simulink model "DHS_Direct_Control_PI"  (R2019b)
settings: Solver=VariableStepAuto  StartTime=0.0  StopTime=0.5  RelTol=1e-3
undefined symbols (not defined in the file): Apd_i_dhs, Apd_u_dhs, C_dhs, f_sw_dhs, L_dhs, Tid_i_dhs, Tid_u_dhs, U_DC
libraries: simulink x2
settings Model: Creator=kissd  LastModifiedBy=kissd

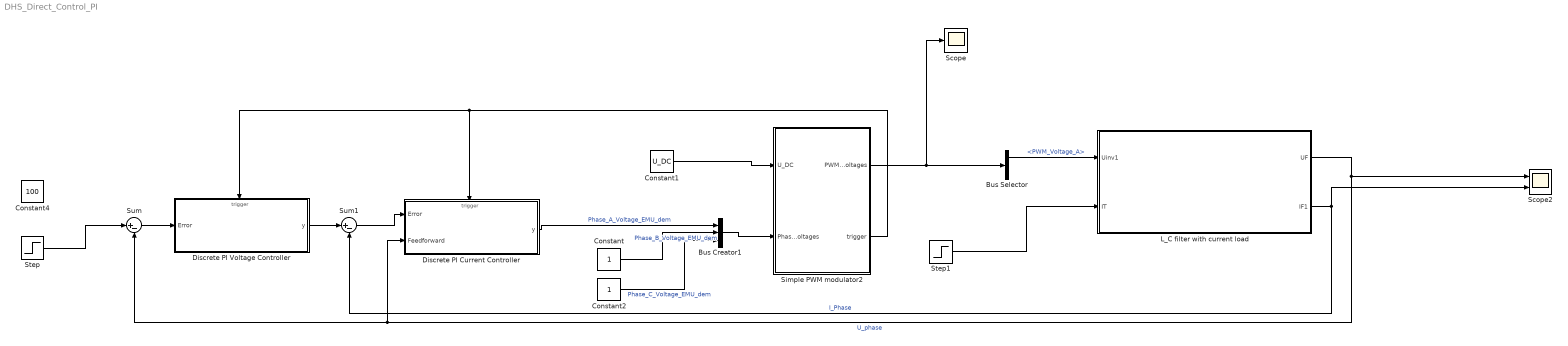
== system DHS_Direct_Control_PI ==
  Bus Creator1 : BusCreator  Inputs=3
  Bus Selector : BusSelector  OutputSignals=PWM_Voltage_A,PWM_Voltage_B,PWM_Voltage_C
  Constant : Constant
  Constant1 : Constant  Value=U_DC
  Constant2 : Constant
  Constant4 : Constant  Value=100
  Discrete PI Current Controller : Subsystem  AncestorBlock=controllers/Discrete PI Controller  mask(Continous PI Controller){Apd=Apd_i_dhs, Tid=Tid_i_dhs, fs=f_sw_dhs, UpperSat=U_DC, LowerSat=0}
      mask prompts: Apd "Proprotional Gain"; Tid "Integration Time"; fs "fsw"; UpperSat "Max. Saturation"; LowerSat "Min. Saturation"
      mask help: Continous PI Controller description.
  Discrete PI Voltage Controller : Subsystem  AncestorBlock=controllers/Discrete PI Controller  mask(Continous PI Controller){Apd=Apd_u_dhs, Tid=Tid_u_dhs, fs=f_sw_dhs, UpperSat=200, LowerSat=-200}
      mask prompts: Apd "Proprotional Gain"; Tid "Integration Time"; fs "fsw"; UpperSat "Max. Saturation"; LowerSat "Min. Saturation"
      mask help: Continous PI Controller description.
  L_C filter with current load : Subsystem
  Scope : Scope
  Scope2 : Scope  NumInputPorts=2
  Simple PWM modulator2 : Subsystem  AncestorBlock=controllers/Simple PWM modulator
  Step : Step  Time=0.2  Before=10  After=200  SampleTime=0
  Step1 : Step  Time=0.3  After=100  SampleTime=0
  Sum : Sum  Inputs=|+-
  Sum1 : Sum  Inputs=|+-
  wires:
  Simple PWM modulator2/2(trigger) -> Discrete PI Voltage Controller/Trigger, Discrete PI Current Controller/Trigger
  Discrete PI Current Controller/1(y) -> Bus Creator1/1  "Phase_A_Voltage_EMU_dem"
  Bus Creator1/1 -> Simple PWM modulator2/2(Phase_Voltages)
  Discrete PI Voltage Controller/1(y) -> Sum1/1
  Step/1 -> Sum/1
  Simple PWM modulator2/1(PWM_Voltages) -> Bus Selector/1, Scope/1
  Sum/1 -> Discrete PI Voltage Controller/1(Error)
  Constant/1 -> Bus Creator1/2  "Phase_B_Voltage_EMU_dem"
  Constant2/1 -> Bus Creator1/3  "Phase_C_Voltage_EMU_dem"
  L_C filter with current load/2(IF1) -> Scope2/2, Sum1/2  "I_Phase"
  L_C filter with current load/1(UF) -> Discrete PI Current Controller/2(Feedforward), Sum/2, Scope2/1  "U_phase"
  Bus Selector/1 -> L_C filter with current load/1(Uinv1)  "<PWM_Voltage_A>"
  Sum1/1 -> Discrete PI Current Controller/1(Error)
  Constant1/1 -> Simple PWM modulator2/1(U_DC)
  Step1/1 -> L_C filter with current load/2(IT)

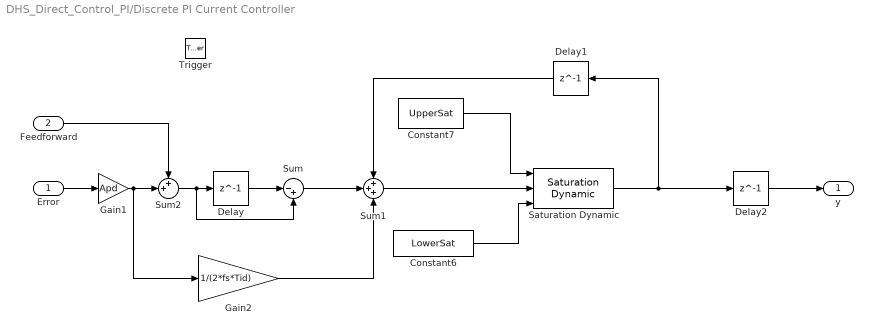
== system DHS_Direct_Control_PI/Discrete PI Current Controller ==
  Error : Inport
  Feedforward : Inport  Port=2
  Trigger : TriggerPort  TriggerType=either  VariantControl=Variant  PortDimensions=1
  Constant6 : Constant  Value=LowerSat
  Constant7 : Constant  Value=UpperSat
  Delay : Delay  DelayLength=1
  Delay1 : Delay  DelayLength=1
  Delay2 : Delay  DelayLength=1
  Gain1 : Gain  Gain=Apd
  Gain2 : Gain  Gain=1/(2*fs*Tid)
  Saturation Dynamic : simulink/Discontinuities/Saturation Dynamic  OutMin=[]  OutMax=[]  OutDataTypeStr=Inherit: Same as second input  OutDataType=fixdt(1, 16)  OutScaling=2^-10  DoSatur=off
  Sum : Sum  Inputs=|-+
  Sum1 : Sum  Inputs=+++
  Sum2 : Sum  Inputs=++|
  y : Outport
  wires:
  Error/1 -> Gain1/1
  Gain1/1 -> Sum2/2, Gain2/1
  Sum1/1 -> Saturation Dynamic/2
  Saturation Dynamic/1 -> Delay1/1, Delay2/1
  Constant7/1 -> Saturation Dynamic/1
  Constant6/1 -> Saturation Dynamic/3
  Delay/1 -> Sum/1
  Sum/1 -> Sum1/2
  Gain2/1 -> Sum1/3
  Delay1/1 -> Sum1/1
  Delay2/1 -> y/1
  Sum2/1 -> Sum/2, Delay/1
  Feedforward/1 -> Sum2/1

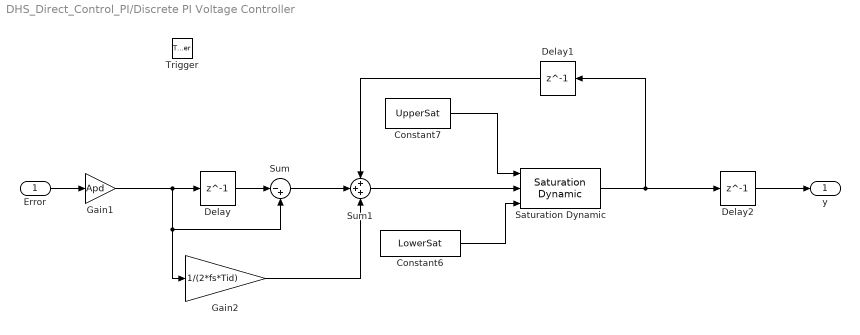
== system DHS_Direct_Control_PI/Discrete PI Voltage Controller ==
  Error : Inport
  Trigger : TriggerPort  TriggerType=either  VariantControl=Variant  PortDimensions=1
  Constant6 : Constant  Value=LowerSat
  Constant7 : Constant  Value=UpperSat
  Delay : Delay  DelayLength=1
  Delay1 : Delay  DelayLength=1
  Delay2 : Delay  DelayLength=1
  Gain1 : Gain  Gain=Apd
  Gain2 : Gain  Gain=1/(2*fs*Tid)
  Saturation Dynamic : simulink/Discontinuities/Saturation Dynamic  OutMin=[]  OutMax=[]  OutDataTypeStr=Inherit: Same as second input  OutDataType=fixdt(1, 16)  OutScaling=2^-10  DoSatur=off
  Sum : Sum  Inputs=|-+
  Sum1 : Sum  Inputs=+++
  y : Outport
  wires:
  Error/1 -> Gain1/1
  Gain1/1 -> Gain2/1, Sum/2, Delay/1
  Sum1/1 -> Saturation Dynamic/2
  Saturation Dynamic/1 -> Delay1/1, Delay2/1
  Constant7/1 -> Saturation Dynamic/1
  Constant6/1 -> Saturation Dynamic/3
  Delay/1 -> Sum/1
  Sum/1 -> Sum1/2
  Gain2/1 -> Sum1/3
  Delay1/1 -> Sum1/1
  Delay2/1 -> y/1

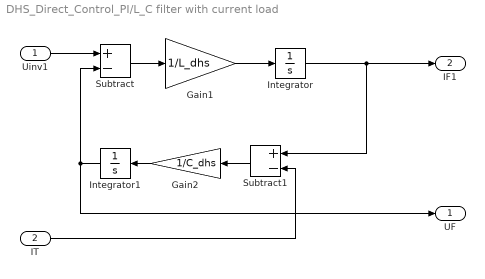
== system DHS_Direct_Control_PI/L_C filter with current load ==
  Uinv1 : Inport
  IT : Inport  Port=2
  Gain1 : Gain  Gain=1/L_dhs
  Gain2 : Gain  Gain=1/C_dhs
  Integrator : Integrator
  Integrator1 : Integrator
  Subtract : Sum  Inputs=+-
  Subtract1 : Sum  Inputs=+-
  UF : Outport
  IF1 : Outport  Port=2
  wires:
  Integrator1/1 -> UF/1, Subtract/2
  Subtract/1 -> Gain1/1
  Gain1/1 -> Integrator/1
  Integrator/1 -> Subtract1/1, IF1/1
  IT/1 -> Subtract1/2
  Gain2/1 -> Integrator1/1
  Uinv1/1 -> Subtract/1
  Subtract1/1 -> Gain2/1

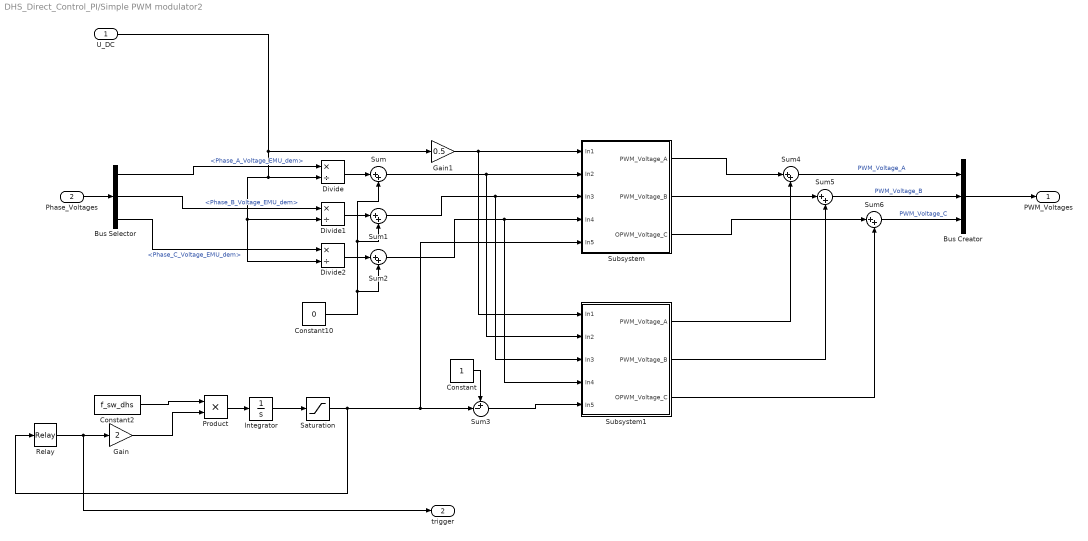
== system DHS_Direct_Control_PI/Simple PWM modulator2 ==
  U_DC : Inport
  Phase_Voltages : Inport  Port=2
  Bus Creator : BusCreator  Inputs=3
  Bus Selector : BusSelector  OutputSignals=Phase_A_Voltage_EMU_dem,Phase_B_Voltage_EMU_dem,Phase_C_Voltage_EMU_dem
  Constant : Constant
  Constant10 : Constant  Value=0
  Constant2 : Constant  Value=f_sw_dhs
  Divide : Product  Inputs=*/
  Divide1 : Product  Inputs=*/
  Divide2 : Product  Inputs=*/
  Gain : Gain  Gain=2
  Gain1 : Gain  Gain=0.5
  Integrator : Integrator
  Product : Product
  Relay : Relay  OnSwitchValue=1  OffSwitchValue=0  OnOutputValue=-1  OffOutputValue=1
  Saturation : Saturate  UpperLimit=1  LowerLimit=0
  Subsystem : Subsystem
  Subsystem1 : Subsystem
  Sum{,1..2,4..6} (6 alike) : Sum  Inputs=|++
  Sum3 : Sum  Inputs=+-|
  PWM_Voltages : Outport
  trigger : Outport  Port=2
  wires:
  Constant2/1 -> Product/1
  Product/1 -> Integrator/1
  Integrator/1 -> Saturation/1
  Divide1/1 -> Sum1/1
  Saturation/1 -> Subsystem/5(In5), Sum3/2, Relay/1
  Relay/1 -> trigger/1, Gain/1
  Constant10/1 -> Sum2/2, Sum1/2, Sum/2
  Bus Selector/1 -> Divide/1  "<Phase_A_Voltage_EMU_dem>"
  Gain/1 -> Product/2
  Divide2/1 -> Sum2/1
  Divide/1 -> Sum/1
  Bus Selector/3 -> Divide2/1  "<Phase_C_Voltage_EMU_dem>"
  Bus Selector/2 -> Divide1/1  "<Phase_B_Voltage_EMU_dem>"
  Phase_Voltages/1 -> Bus Selector/1
  Bus Creator/1 -> PWM_Voltages/1
  Constant/1 -> Sum3/1
  Sum/1 -> Subsystem1/2(In2), Subsystem/2(In2)
  Sum1/1 -> Subsystem1/3(In3), Subsystem/3(In3)
  Sum2/1 -> Subsystem1/4(In4), Subsystem/4(In4)
  Sum3/1 -> Subsystem1/5(In5)
  Sum4/1 -> Bus Creator/1  "PWM_Voltage_A"
  Subsystem/1(PWM_Voltage_A) -> Sum4/1
  Subsystem1/1(PWM_Voltage_A) -> Sum4/2
  Sum5/1 -> Bus Creator/2  "PWM_Voltage_B"
  Subsystem/2(PWM_Voltage_B) -> Sum5/1
  Subsystem1/2(PWM_Voltage_B) -> Sum5/2
  Sum6/1 -> Bus Creator/3  "PWM_Voltage_C"
  Subsystem/3(OPWM_Voltage_C) -> Sum6/1
  Subsystem1/3(OPWM_Voltage_C) -> Sum6/2
  U_DC/1 -> Gain1/1, Divide2/2, Divide1/2, Divide/2
  Gain1/1 -> Subsystem1/1(In1), Subsystem/1(In1)

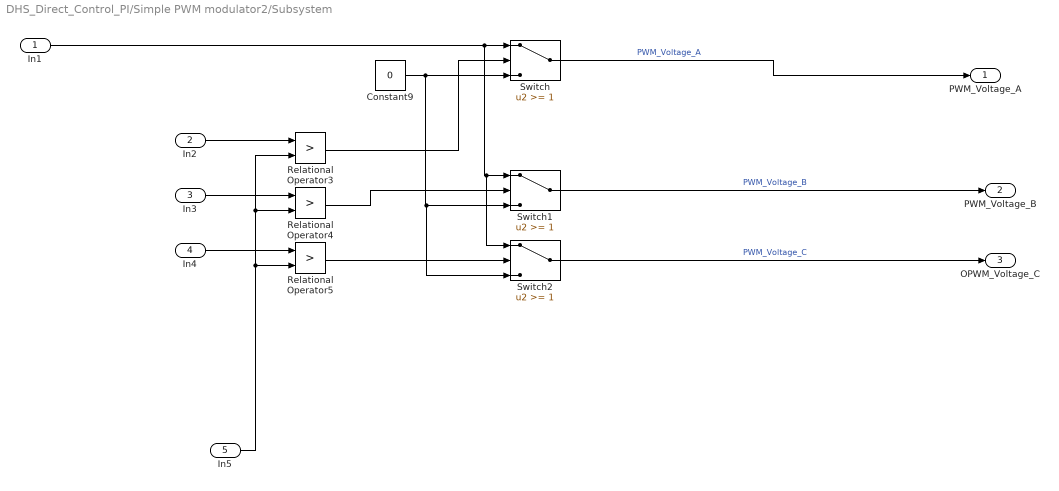
== system DHS_Direct_Control_PI/Simple PWM modulator2/Subsystem ==
  In1 : Inport
  In2 : Inport  Port=2
  In3 : Inport  Port=3
  In4 : Inport  Port=4
  In5 : Inport  Port=5
  Constant9 : Constant  Value=0
  Relational Operator3 : RelationalOperator  Operator=>  OutDataTypeStr=boolean  RndMeth=Simplest
  Relational Operator4 : RelationalOperator  Operator=>  OutDataTypeStr=boolean  RndMeth=Simplest
  Relational Operator5 : RelationalOperator  Operator=>  OutDataTypeStr=boolean  RndMeth=Simplest
  Switch : Switch  Threshold=1
  Switch1 : Switch  Threshold=1
  Switch2 : Switch  Threshold=1
  PWM_Voltage_A : Outport
  PWM_Voltage_B : Outport  Port=2
  OPWM_Voltage_C : Outport  Port=3
  wires:
  Relational Operator4/1 -> Switch1/2
  In5/1 -> Relational Operator3/2, Relational Operator4/2, Relational Operator5/2
  Constant9/1 -> Switch2/3, Switch1/3, Switch/3
  Relational Operator3/1 -> Switch/2
  In3/1 -> Relational Operator4/1
  Relational Operator5/1 -> Switch2/2
  Switch/1 -> PWM_Voltage_A/1  "PWM_Voltage_A"
  In1/1 -> Switch2/1, Switch1/1, Switch/1
  In2/1 -> Relational Operator3/1
  In4/1 -> Relational Operator5/1
  Switch1/1 -> PWM_Voltage_B/1  "PWM_Voltage_B"
  Switch2/1 -> OPWM_Voltage_C/1  "PWM_Voltage_C"

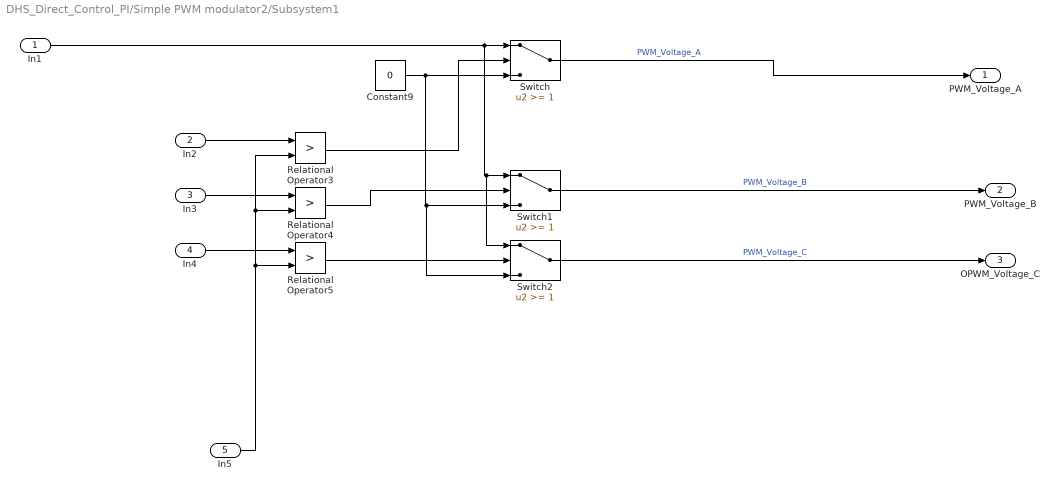
== system DHS_Direct_Control_PI/Simple PWM modulator2/Subsystem1 ==
  In1 : Inport
  In2 : Inport  Port=2
  In3 : Inport  Port=3
  In4 : Inport  Port=4
  In5 : Inport  Port=5
  Constant9 : Constant  Value=0
  Relational Operator3 : RelationalOperator  Operator=>  OutDataTypeStr=boolean  RndMeth=Simplest
  Relational Operator4 : RelationalOperator  Operator=>  OutDataTypeStr=boolean  RndMeth=Simplest
  Relational Operator5 : RelationalOperator  Operator=>  OutDataTypeStr=boolean  RndMeth=Simplest
  Switch : Switch  Threshold=1
  Switch1 : Switch  Threshold=1
  Switch2 : Switch  Threshold=1
  PWM_Voltage_A : Outport
  PWM_Voltage_B : Outport  Port=2
  OPWM_Voltage_C : Outport  Port=3
  wires:
  Relational Operator4/1 -> Switch1/2
  In5/1 -> Relational Operator3/2, Relational Operator4/2, Relational Operator5/2
  Constant9/1 -> Switch2/3, Switch1/3, Switch/3
  Relational Operator3/1 -> Switch/2
  In3/1 -> Relational Operator4/1
  Relational Operator5/1 -> Switch2/2
  Switch/1 -> PWM_Voltage_A/1  "PWM_Voltage_A"
  In1/1 -> Switch2/1, Switch1/1, Switch/1
  In2/1 -> Relational Operator3/1
  In4/1 -> Relational Operator5/1
  Switch1/1 -> PWM_Voltage_B/1  "PWM_Voltage_B"
  Switch2/1 -> OPWM_Voltage_C/1  "PWM_Voltage_C"
